simulink model "Six_phase_inverter_double"  (R2014b)
settings: Solver=ode23tb  StartTime=0.0  StopTime=0.05  MaxStep=1e-4  RelTol=1e-3
InitFcn:
  | Vm=0.5;
  | Fc=3000;
libraries: powerlib x12, simulink x1
settings Model: Creator=y  LastModifiedBy=Lei
settings DataIOCC: SignalLoggingSaveFormat=ModelDataLogs
settings OptimizationCC: ExpressionDepthLimit=2147483647  InitFltsAndDblsToZero=on
settings DebuggingCC: SaveWithParameterizedLinksMsg=none  UnderspecifiedInitializationDetection=Classic  MergeDetectMultiDrivingBlocksExec=none  SignalResolutionControl=TryResolveAllWithWarning  MultiTaskDSMMsg=warning  MultiTaskCondExecSysMsg=none  FcnCallInpInsideContextMsg=UseLocalSettings  StateNameClashWarn=warning
settings RTWCC: IncludeERTFirstTime=on
settings GRTTargetCC: TargetFcnLib=ansi_tfl_tmw.mat  CombineOutputUpdateFcns=off  GRTInterface=on

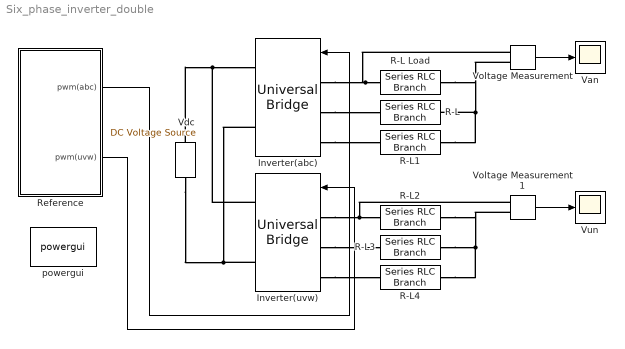
== system Six_phase_inverter_double ==
  Inverter(abc) : powerlib/Power Electronics/Universal Bridge  Arms=3  SnubberResistance=1e5  SnubberCapacitance=inf  Device=IGBT / Diodes  Ron=1e-3  Lon=0  ForwardVoltages="[  0  0  ]"  ForwardVoltage=0  GTOparameters=[ 10e-6 , 20e-6 ]  IGBTparameters=[ 1e-6 , 2e-6 ]  Measurements=None  Measurements_2=None  converterType=Rectifier
  Inverter(uvw) : powerlib/Power Electronics/Universal Bridge  Arms=3  SnubberResistance=1e5  SnubberCapacitance=inf  Device=IGBT / Diodes  Ron=1e-3  Lon=0  ForwardVoltages="[  0  0  ]"  ForwardVoltage=0  GTOparameters=[ 10e-6 , 20e-6 ]  IGBTparameters=[ 1e-6 , 2e-6 ]  Measurements=None  Measurements_2=None  converterType=Rectifier
  R-L{,1..4} (5 alike) : powerlib/Elements/Series RLC Branch  LConnTagsString=__new0  RConnTagsString=__new0  BranchType=RL  Resistance=10  Inductance=1e-03  SetiL0=off  InitialCurrent=0  Capacitance=[]  Setx0=off  InitialVoltage=0  Measurements=None
  R-L Load : powerlib/Elements/Series RLC Branch  LConnTagsString=__new0  RConnTagsString=__new0  BranchType=RL  Resistance=10  Inductance=1e-03  SetiL0=off  InitialCurrent=0  Capacitance=[]  Setx0=off  InitialVoltage=0  Measurements=None
  Reference : Subsystem
  Van : Scope
      settings: TimeRange=0.05  YMin=-200  YMax=200  SaveName=Van  SampleInput=on  SampleTime=1e-6
  Vdc : powerlib/Electrical Sources/DC Voltage Source  Amplitude=300  Measurements=None
  Voltage Measurement : powerlib/Measurements/Voltage Measurement  PhasorSimulation=off  OutputType=Complex  PSBequivalent=0
  Voltage Measurement1 : powerlib/Measurements/Voltage Measurement  PhasorSimulation=off  OutputType=Complex  PSBequivalent=0
  Vun : Scope
      settings: YMin=-200  YMax=200  SaveName=Vbn  SampleInput=on  SampleTime=1e-6
  powergui : powerlib/powergui  Priority=1  SimulationMode=Continuous  SolverType=Tustin/Backward Euler (TBE)  SampleTime=50e-6  frequency=60  SPID=off  DisableSnubberDevices=off  DisableRonSwitches=off  DisableVfSwitches=off  SwTol=0  DisplayEquations=off  Interpol=off  methode=off  Ts=100  frequencyindice=0  Pbase=100e6  ErrMax=1e-4  Iterations=50  UnitsV=kV  UnitsW=MW  FunctionMessages=off  echomessages=off  HookPort=off  EnableUseOfTLC=off  x0status=blocks  RestoreLinks=warning  ResistiveCurrentMeasurement=off  Frange=[0:2:500]  Ylog=off  Xlog=on  ShowGrid=off  save=off  variable=ZData  structure=0  ZoomFFT=off  StartTime=0.0  cycles=1  DisplayStyle=1  fundamental=60  FreqAxis=off  MaxFrequency=1000  frequencyindicesteady=1  RmsSteady=1  display=off
  wires:
  Voltage Measurement/1 -> Van/1
  Voltage Measurement1/1 -> Vun/1
  Reference/1(pwm(abc)) -> Inverter(abc)/1
  Reference/2(pwm(uvw)) -> Inverter(uvw)/1
  connections:
  R-L Load/LConn1 -- Inverter(abc)/LConn1 -- Voltage Measurement/LConn1
  Inverter(abc)/LConn2 -- R-L/LConn1
  Inverter(abc)/LConn3 -- R-L1/LConn1
  Voltage Measurement1/LConn1 -- Inverter(uvw)/LConn1 -- R-L2/LConn1
  Inverter(uvw)/LConn2 -- R-L3/LConn1
  Inverter(uvw)/LConn3 -- R-L4/LConn1
  R-L4/RConn1 -- Voltage Measurement1/LConn2 -- R-L2/RConn1 -- R-L3/RConn1
  R-L1/RConn1 -- Voltage Measurement/LConn2 -- R-L Load/RConn1 -- R-L/RConn1
  Vdc/RConn1 -- Inverter(uvw)/RConn1 -- Inverter(abc)/RConn1
  Vdc/LConn1 -- Inverter(uvw)/RConn2 -- Inverter(abc)/RConn2

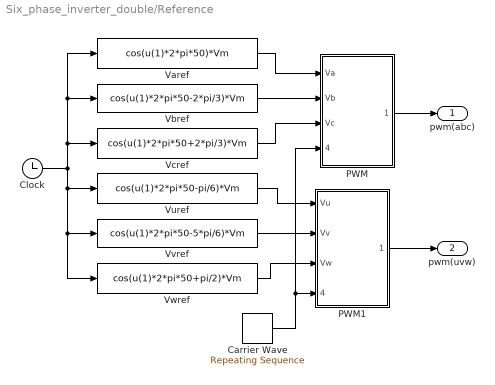
== system Six_phase_inverter_double/Reference ==
  Carrier Wave : simulink/Sources/Repeating Sequence  rep_seq_t=[0 1/Fc/4 3/Fc/4 1/Fc]  rep_seq_y=[0 -1 1 0]
  Clock : Clock
  PWM : Subsystem
  PWM1 : Subsystem
  Varef : Fcn  Expr=cos(u(1)*2*pi*50)*Vm
  Vbref : Fcn  Expr=cos(u(1)*2*pi*50-2*pi/3)*Vm
  Vcref : Fcn  Expr=cos(u(1)*2*pi*50+2*pi/3)*Vm
  Vuref : Fcn  Expr=cos(u(1)*2*pi*50-pi/6)*Vm
  Vvref : Fcn  Expr=cos(u(1)*2*pi*50-5*pi/6)*Vm
  Vwref : Fcn  Expr=cos(u(1)*2*pi*50+pi/2)*Vm
  pwm(abc) : Outport
  pwm(uvw) : Outport  Port=2
  wires:
  Clock/1 -> Varef/1, Vbref/1, Vcref/1, Vwref/1, Vvref/1, Vuref/1
  Varef/1 -> PWM/1(Va)
  Vbref/1 -> PWM/2(Vb)
  Vcref/1 -> PWM/3(Vc)
  Vvref/1 -> PWM1/2(Vv)
  Vwref/1 -> PWM1/3(Vw)
  Vuref/1 -> PWM1/1(Vu)
  Carrier Wave/1 -> PWM1/4(Carrier wave), PWM/4(Carrier wave)
  PWM/1(pwm(abc)) -> pwm(abc)/1
  PWM1/1(pwm(uvw)) -> pwm(uvw)/1

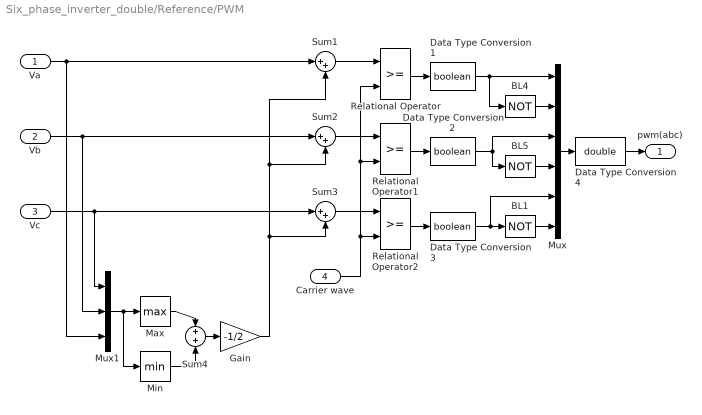
== system Six_phase_inverter_double/Reference/PWM ==
  Va : Inport
  Vb : Inport  Port=2
  Vc : Inport  Port=3
  Carrier wave : Inport  Port=4
  BL1 : Logic  Operator=NOT  Inputs=1
  BL4 : Logic  Operator=NOT  Inputs=1
  BL5 : Logic  Operator=NOT  Inputs=1
  Data Type Conversion1 : DataTypeConversion  OutDataTypeStr=boolean  SaturateOnIntegerOverflow=on  RndMeth=Zero
  Data Type Conversion2 : DataTypeConversion  OutDataTypeStr=boolean  SaturateOnIntegerOverflow=on  RndMeth=Zero
  Data Type Conversion3 : DataTypeConversion  OutDataTypeStr=boolean  SaturateOnIntegerOverflow=on  RndMeth=Zero
  Data Type Conversion4 : DataTypeConversion  OutDataTypeStr=double  SaturateOnIntegerOverflow=on  RndMeth=Zero
  Gain : Gain  Gain=-1/2
  Max : MinMax  Function=max
  Min : MinMax
  Mux : Mux  Inputs=6
  Mux1 : Mux  Inputs=3
  Relational Operator : RelationalOperator  InputSameDT=on
  Relational Operator1 : RelationalOperator  InputSameDT=on
  Relational Operator2 : RelationalOperator  InputSameDT=on
  Sum1 : Sum  Inputs=|++
  Sum2 : Sum  Inputs=|++
  Sum3 : Sum  Inputs=|++
  Sum4 : Sum  Inputs=+|+
  pwm(abc) : Outport
  wires:
  Carrier wave/1 -> Relational Operator1/2, Relational Operator/2, Relational Operator2/2
  Data Type Conversion1/1 -> Mux/1, BL4/1
  Relational Operator/1 -> Data Type Conversion1/1
  Data Type Conversion2/1 -> BL5/1, Mux/3
  Relational Operator1/1 -> Data Type Conversion2/1
  BL4/1 -> Mux/2
  BL5/1 -> Mux/4
  BL1/1 -> Mux/6
  Relational Operator2/1 -> Data Type Conversion3/1
  Mux/1 -> Data Type Conversion4/1
  Data Type Conversion4/1 -> pwm(abc)/1
  Va/1 -> Mux1/3, Sum1/1
  Sum1/1 -> Relational Operator/1
  Sum2/1 -> Relational Operator1/1
  Vb/1 -> Mux1/2, Sum2/1
  Vc/1 -> Mux1/1, Sum3/1
  Sum3/1 -> Relational Operator2/1
  Mux1/1 -> Min/1, Max/1
  Data Type Conversion3/1 -> Mux/5, BL1/1
  Min/1 -> Sum4/2
  Max/1 -> Sum4/1
  Sum4/1 -> Gain/1
  Gain/1 -> Sum2/2, Sum1/2, Sum3/2

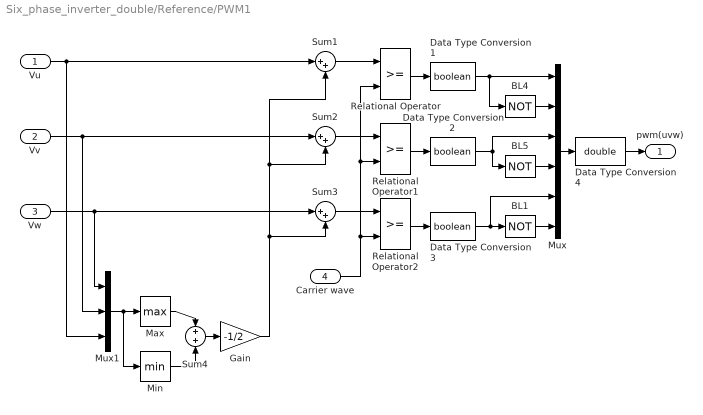
== system Six_phase_inverter_double/Reference/PWM1 ==
  Vu : Inport
  Vv : Inport  Port=2
  Vw : Inport  Port=3
  Carrier wave : Inport  Port=4
  BL1 : Logic  Operator=NOT  Inputs=1
  BL4 : Logic  Operator=NOT  Inputs=1
  BL5 : Logic  Operator=NOT  Inputs=1
  Data Type Conversion1 : DataTypeConversion  OutDataTypeStr=boolean  SaturateOnIntegerOverflow=on  RndMeth=Zero
  Data Type Conversion2 : DataTypeConversion  OutDataTypeStr=boolean  SaturateOnIntegerOverflow=on  RndMeth=Zero
  Data Type Conversion3 : DataTypeConversion  OutDataTypeStr=boolean  SaturateOnIntegerOverflow=on  RndMeth=Zero
  Data Type Conversion4 : DataTypeConversion  OutDataTypeStr=double  SaturateOnIntegerOverflow=on  RndMeth=Zero
  Gain : Gain  Gain=-1/2
  Max : MinMax  Function=max
  Min : MinMax
  Mux : Mux  Inputs=6
  Mux1 : Mux  Inputs=3
  Relational Operator : RelationalOperator  InputSameDT=on
  Relational Operator1 : RelationalOperator  InputSameDT=on
  Relational Operator2 : RelationalOperator  InputSameDT=on
  Sum1 : Sum  Inputs=|++
  Sum2 : Sum  Inputs=|++
  Sum3 : Sum  Inputs=|++
  Sum4 : Sum  Inputs=+|+
  pwm(uvw) : Outport
  wires:
  Gain/1 -> Sum3/2, Sum1/2, Sum2/2
  Sum4/1 -> Gain/1
  Max/1 -> Sum4/1
  Min/1 -> Sum4/2
  Data Type Conversion3/1 -> BL1/1, Mux/5
  Mux1/1 -> Max/1, Min/1
  Sum3/1 -> Relational Operator2/1
  Vw/1 -> Sum3/1, Mux1/1
  Vv/1 -> Sum2/1, Mux1/2
  Sum2/1 -> Relational Operator1/1
  Sum1/1 -> Relational Operator/1
  Vu/1 -> Sum1/1, Mux1/3
  Data Type Conversion4/1 -> pwm(uvw)/1
  Mux/1 -> Data Type Conversion4/1
  Relational Operator2/1 -> Data Type Conversion3/1
  BL1/1 -> Mux/6
  BL5/1 -> Mux/4
  BL4/1 -> Mux/2
  Relational Operator1/1 -> Data Type Conversion2/1
  Data Type Conversion2/1 -> Mux/3, BL5/1
  Relational Operator/1 -> Data Type Conversion1/1
  Data Type Conversion1/1 -> BL4/1, Mux/1
  Carrier wave/1 -> Relational Operator2/2, Relational Operator/2, Relational Operator1/2
